simulink model "x3otu"  (R2023a)
settings: Solver=VariableStepAuto  StartTime=0.0  StopTime=500  RelTol=1e-3
settings Model: Creator=etoki  LastModifiedBy=etoki
settings SolverCC: ZeroCrossAlgorithm=Adaptive
settings DebuggingCC: IgnoredZcDiagnostic=none

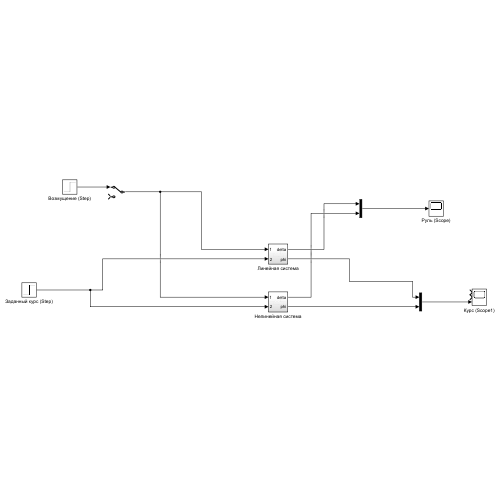
[thumbnail: Simulink's stored preview of the top-level diagram]
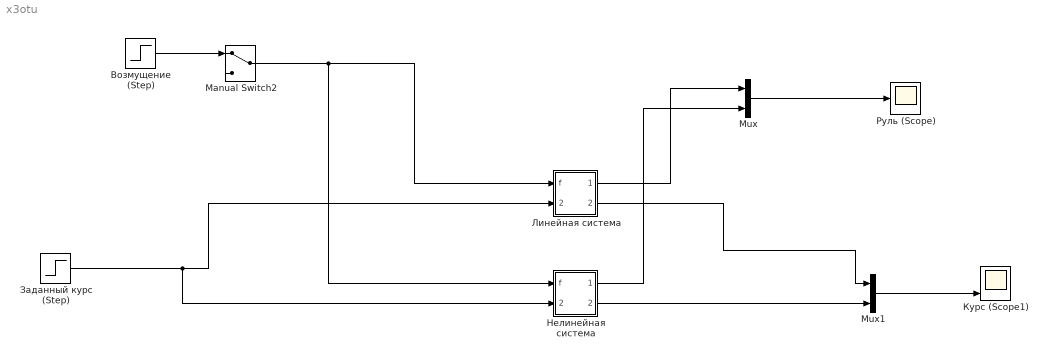
== system x3otu ==
  Manual Switch2 : ManualSwitch
  Mux : Mux  Inputs=2
  Mux1 : Mux  Inputs=2
  Возмущение (Step) : Step  SampleTime=0
  Заданный курс (Step) : Step  Time=0  After=90  SampleTime=0
  Курс (Scope1) : Scope  NumInputPorts=3
  Линейная система : Subsystem
  Нелинейная система : Subsystem
  Руль (Scope) : Scope
  wires:
  Заданный курс (Step)/1 -> Нелинейная система/2(In2), Линейная система/2(In2)
  Возмущение (Step)/1 -> Manual Switch2/1
  Manual Switch2/1 -> Нелинейная система/1(f), Линейная система/1(f)
  Линейная система/1(delta) -> Mux/1
  Линейная система/2(phi) -> Mux1/1
  Нелинейная система/2(phi) -> Mux1/2
  Mux/1 -> Руль (Scope)/1
  Mux1/1 -> Курс (Scope1)/3
  Нелинейная система/1(delta) -> Mux/2

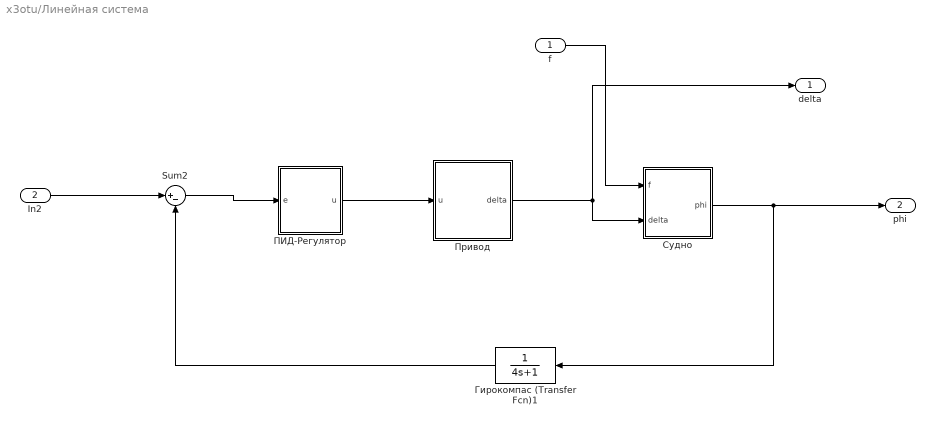
== system x3otu/Линейная система ==
  f : Inport
  In2 : Inport  Port=2
  Sum2 : Sum  Inputs=|+-
  Гирокомпас (Transfer Fcn)1 : TransferFcn  Denominator=[4 1]
  ПИД-Регулятор : Subsystem
  Привод : Subsystem
  Судно : Subsystem
  delta : Outport
  phi : Outport  Port=2
  wires:
  Судно/1(phi) -> phi/1, Гирокомпас (Transfer Fcn)1/1
  Sum2/1 -> ПИД-Регулятор/1(e)
  Гирокомпас (Transfer Fcn)1/1 -> Sum2/2
  Привод/1(delta) -> delta/1, Судно/2(delta)
  ПИД-Регулятор/1(u) -> Привод/1(u)
  In2/1 -> Sum2/1
  f/1 -> Судно/1(f)

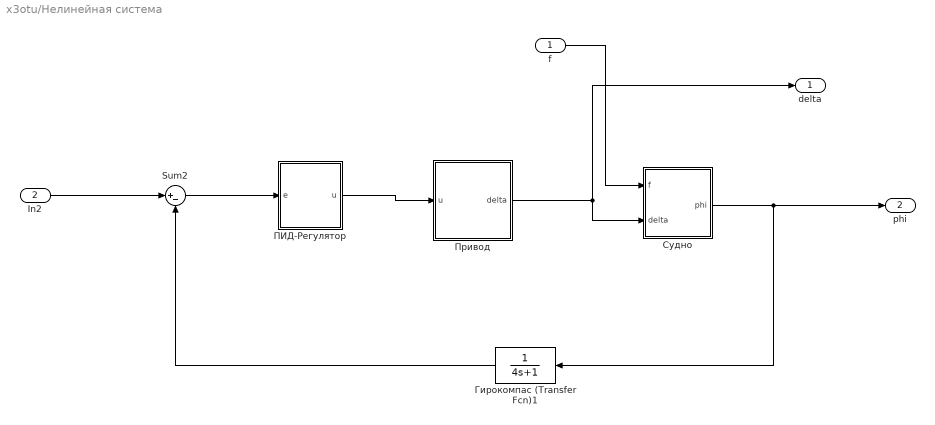
== system x3otu/Нелинейная система ==
  f : Inport
  In2 : Inport  Port=2
  Sum2 : Sum  Inputs=|+-
  Гирокомпас (Transfer Fcn)1 : TransferFcn  Denominator=[4 1]
  ПИД-Регулятор : Subsystem
  Привод : Subsystem
  Судно : Subsystem
  delta : Outport
  phi : Outport  Port=2
  wires:
  Судно/1(phi) -> phi/1, Гирокомпас (Transfer Fcn)1/1
  Sum2/1 -> ПИД-Регулятор/1(e)
  Гирокомпас (Transfer Fcn)1/1 -> Sum2/2
  Привод/1(delta) -> delta/1, Судно/2(delta)
  ПИД-Регулятор/1(u) -> Привод/1(u)
  In2/1 -> Sum2/1
  f/1 -> Судно/1(f)

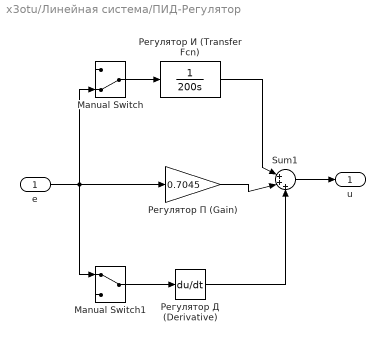
== system x3otu/Линейная система/ПИД-Регулятор ==
  e : Inport
  Manual Switch : ManualSwitch  CurrentSetting=0
  Manual Switch1 : ManualSwitch
  Sum1 : Sum  Inputs=|+++
  Регулятор Д (Derivative) : Derivative
  Регулятор И (Transfer Fcn) : TransferFcn  Denominator=[200 0]
  Регулятор П (Gain) : Gain  Gain=0.7045
  u : Outport
  wires:
  e/1 -> Manual Switch1/1, Manual Switch/2, Регулятор П (Gain)/1
  Регулятор И (Transfer Fcn)/1 -> Sum1/1
  Регулятор Д (Derivative)/1 -> Sum1/3
  Sum1/1 -> u/1
  Manual Switch1/1 -> Регулятор Д (Derivative)/1
  Manual Switch/1 -> Регулятор И (Transfer Fcn)/1
  Регулятор П (Gain)/1 -> Sum1/2

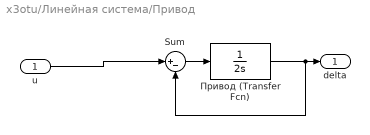
== system x3otu/Линейная система/Привод ==
  u : Inport
  Sum : Sum  Inputs=|+-
  Привод (Transfer Fcn) : TransferFcn  Denominator=[2 0]
  delta : Outport
  wires:
  Sum/1 -> Привод (Transfer Fcn)/1
  Привод (Transfer Fcn)/1 -> Sum/2, delta/1
  u/1 -> Sum/1

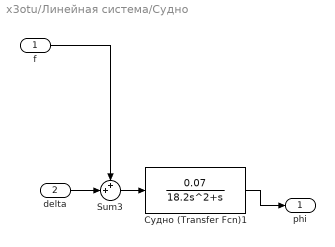
== system x3otu/Линейная система/Судно ==
  f : Inport
  delta : Inport  Port=2
  Sum3 : Sum  Inputs=++|
  Судно (Transfer Fcn)1 : TransferFcn  Numerator=[0.07]  Denominator=[18.2 1 0]
  phi : Outport
  wires:
  Sum3/1 -> Судно (Transfer Fcn)1/1
  delta/1 -> Sum3/2
  f/1 -> Sum3/1
  Судно (Transfer Fcn)1/1 -> phi/1

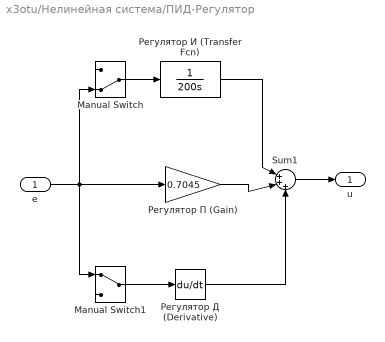
== system x3otu/Нелинейная система/ПИД-Регулятор ==
  e : Inport
  Manual Switch : ManualSwitch  CurrentSetting=0
  Manual Switch1 : ManualSwitch
  Sum1 : Sum  Inputs=|+++
  Регулятор Д (Derivative) : Derivative
  Регулятор И (Transfer Fcn) : TransferFcn  Denominator=[200 0]
  Регулятор П (Gain) : Gain  Gain=0.7045
  u : Outport
  wires:
  e/1 -> Manual Switch1/1, Manual Switch/2, Регулятор П (Gain)/1
  Регулятор И (Transfer Fcn)/1 -> Sum1/1
  Регулятор Д (Derivative)/1 -> Sum1/3
  Sum1/1 -> u/1
  Manual Switch1/1 -> Регулятор Д (Derivative)/1
  Manual Switch/1 -> Регулятор И (Transfer Fcn)/1
  Регулятор П (Gain)/1 -> Sum1/2

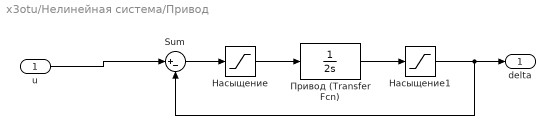
== system x3otu/Нелинейная система/Привод ==
  u : Inport
  Sum : Sum  Inputs=|+-
  Насыщение : Saturate  UpperLimit=3  LowerLimit=-3
  Насыщение1 : Saturate  UpperLimit=50  LowerLimit=-50
  Привод (Transfer Fcn) : TransferFcn  Denominator=[2 0]
  delta : Outport
  wires:
  Sum/1 -> Насыщение/1
  Привод (Transfer Fcn)/1 -> Насыщение1/1
  u/1 -> Sum/1
  Насыщение/1 -> Привод (Transfer Fcn)/1
  Насыщение1/1 -> Sum/2, delta/1

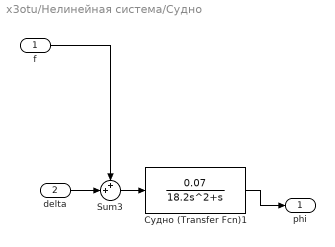
== system x3otu/Нелинейная система/Судно ==
  f : Inport
  delta : Inport  Port=2
  Sum3 : Sum  Inputs=++|
  Судно (Transfer Fcn)1 : TransferFcn  Numerator=[0.07]  Denominator=[18.2 1 0]
  phi : Outport
  wires:
  Sum3/1 -> Судно (Transfer Fcn)1/1
  delta/1 -> Sum3/2
  f/1 -> Sum3/1
  Судно (Transfer Fcn)1/1 -> phi/1
